simulink model "momentumBasedFlying"  (R2021b)
settings: Solver=FixedStepAuto  StartTime=0.0  StopTime=Config.simulationTime  FixedStep=Config.tStep  RelTol=1e-3
InitFcn:
  | cd(fileparts(which(bdroot)));
  | initMomentumBasedFlying;
StopFcn:
  | cd(fileparts(which(bdroot)));
  | stopMomentumBasedFlying;
undefined symbols (not defined in the file or in its folder): biasVectorConstraint_feet, Config, confVisualizer, ConstraintMatrix_feet, DiscIntNeverNeededParam, jets_config
libraries: WBToolboxLibrary x75
(part 1 of 4)
settings Model: NumberOfSteps=50  Creator=gnava  LastModifiedBy=tonhu
settings SolverCC: AlgebraicLoopSolver=LineSearch
settings DataIOCC: ReturnWorkspaceOutputs=off
settings OptimizationCC: BlockReduction=off  DefaultParameterBehavior=Inlined  BufferReuse=off
settings DebuggingCC: PregeneratedLibrarySubsystemCodeDiagnostic=none  SFMachineParentedDataDiag=warning  ArithmeticOperatorsInVariantConditions=warning
settings SFSimCC: SimUseLocalCustomCode=off  CustomCodeUndefinedFunction=UseInterfaceOnly
settings RTWCC: RTWUseLocalCustomCode=off

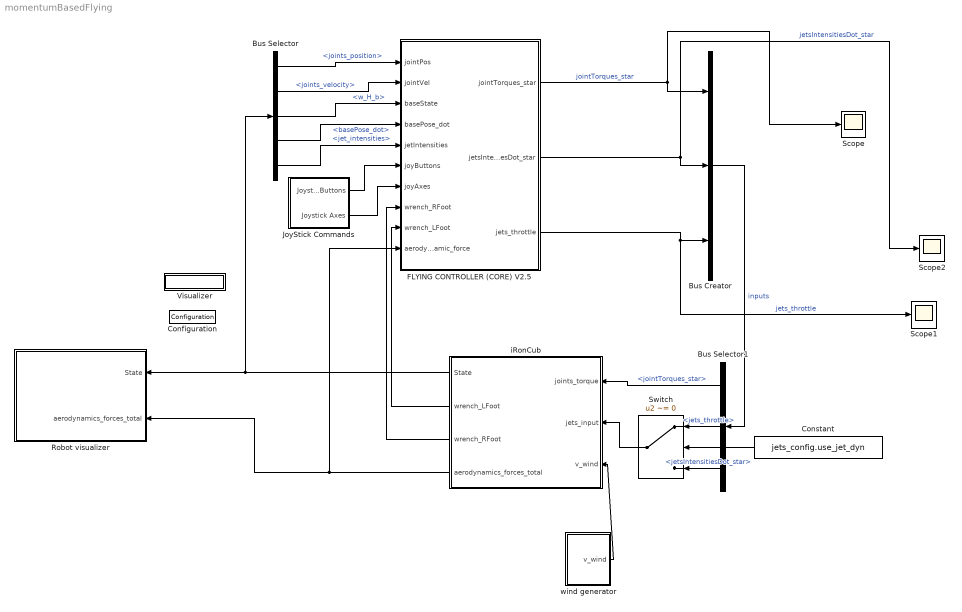
== system momentumBasedFlying ==
  Bus Creator : BusCreator  Inputs=3
  Bus Selector : BusSelector  OutputSignals=joints_position,joints_velocity,w_H_b,basePose_dot,jet_intensities
  Bus Selector1 : BusSelector  OutputSignals=jointTorques_star,jets_throttle,jetsIntensitiesDot_star
  Configuration : WBToolboxLibrary/Utilities/Configuration  ConfigSource=Workspace  ConfigObject='WBTConfigRobot'
      settings: SourceProductName=WholeBodyToolbox
  Constant : Constant  Value=jets_config.use_jet_dyn
  FLYING CONTROLLER (CORE) V2.5 : Subsystem  SystemSampleTime=0.01
  JoyStick Commands : Subsystem
  Robot visualizer : Subsystem  TreatAsAtomicUnit=on  SystemSampleTime=confVisualizer.tStep
  Scope : Scope
  Scope1 : Scope
  Scope2 : Scope
  Switch : Switch  Criteria=u2 ~= 0
  Visualizer : Subsystem
      mask Display: disp('VISUALIZER')
  iRonCub : Subsystem  SystemSampleTime=0.001
  wind generator : Subsystem
  wires:
  JoyStick Commands/1(Joystick Buttons) -> FLYING CONTROLLER (CORE) V2.5/6(joyButtons)
  JoyStick Commands/2(Joystick Axes) -> FLYING CONTROLLER (CORE) V2.5/7(joyAxes)
  iRonCub/1(State) -> Bus Selector/1, Robot visualizer/1(State)
  Bus Selector/1 -> FLYING CONTROLLER (CORE) V2.5/1(jointPos)  "<joints_position>"
  Bus Selector/2 -> FLYING CONTROLLER (CORE) V2.5/2(jointVel)  "<joints_velocity>"
  Bus Selector/3 -> FLYING CONTROLLER (CORE) V2.5/3(baseState)  "<w_H_b>"
  Bus Selector/4 -> FLYING CONTROLLER (CORE) V2.5/4("basePose_dot ")  "<basePose_dot>"
  Bus Selector/5 -> FLYING CONTROLLER (CORE) V2.5/5(jetIntensities)  "<jet_intensities>"
  Bus Creator/1 -> Bus Selector1/1  "inputs"
  FLYING CONTROLLER (CORE) V2.5/2(jetsIntensitiesDot_star) -> Scope2/1, Bus Creator/2  "jetsIntensitiesDot_star"
  FLYING CONTROLLER (CORE) V2.5/1(jointTorques_star) -> Scope/1, Bus Creator/1  "jointTorques_star"
  Bus Selector1/1 -> iRonCub/1(joints_torque)  "<jointTorques_star>"
  FLYING CONTROLLER (CORE) V2.5/3(jets_throttle) -> Scope1/1, Bus Creator/3  "jets_throttle"
  iRonCub/2(wrench_LFoot) -> FLYING CONTROLLER (CORE) V2.5/9(wrench_LFoot)
  iRonCub/3(wrench_RFoot) -> FLYING CONTROLLER (CORE) V2.5/8(wrench_RFoot)
  Switch/1 -> iRonCub/2(jets_input)
  Constant/1 -> Switch/2
  Bus Selector1/2 -> Switch/1  "<jets_throttle>"
  Bus Selector1/3 -> Switch/3  "<jetsIntensitiesDot_star>"
  iRonCub/4(aerodynamics_forces_total) -> FLYING CONTROLLER (CORE) V2.5/10(aerodynamic_force), Robot visualizer/2(aerodynamics_forces_total)
  wind generator/1(v_wind) -> iRonCub/3(v_wind)

== system momentumBasedFlying/FLYING CONTROLLER (CORE) V2.5 ==
  jointPos : Inport
  jointVel : Inport  Port=2
  baseState : Inport  Port=3
  "basePose_dot " : Inport  Port=4
  jetIntensities : Inport  Port=5
  joyButtons : Inport  Port=6
  joyAxes : Inport  Port=7
  wrench_RFoot : Inport  Port=8
  wrench_LFoot : Inport  Port=9
  aerodynamic_force : Inport  Port=10
  Dynamics and Kinematics : Subsystem
  Flight Controller RAL-HUMANOIDS V3.1- Aerodynamic Effects Compensation : Subsystem  mask{Parameter1=Config}
      mask prompts: Parameter1 "Specify the parameters struct"
      mask DialogControl DescGroupVar Prompt: Flight Controller RAL-HUMANOIDS
      mask DialogControl DescTextVar Prompt: This block implements the momentum-based flight controller decribed in RAL 2018 and HUMANOIDS 2018 papers.
      mask DialogControl Control3 Prompt: References:
      mask DialogControl Control5 Prompt: RAL 2018 paper
      mask DialogControl Control5 Callback: web https://ieeexplore.ieee.org/document/7997895
      mask DialogControl Control6 Prompt: HUMANOIDS 2018 paper
      mask DialogControl Control6 Callback: web https://ieeexplore.ieee.org/document/8624985
  Flying State Machine : Subsystem
  Get System State : Subsystem
  jointTorques_star : Outport  VectorParamsAs1DForOutWhenUnconnected=off
  jetsIntensitiesDot_star : Outport  Port=2  VectorParamsAs1DForOutWhenUnconnected=off
  jets_throttle : Outport  Port=3
  wires:
  wrench_LFoot/1 -> Get System State/6(wrench_LFoot)
  Get System State/1(systemState) -> Flight Controller RAL-HUMANOIDS V3.1- Aerodynamic Effects Compensation/3(systemState), Flying State Machine/3(systemState), Dynamics and Kinematics/1(systemState)
  joyButtons/1 -> Flying State Machine/1(joyButtons)
  jetIntensities/1 -> Get System State/7(jetIntensities)
  joyAxes/1 -> Flying State Machine/2(joyAxes)
  jointVel/1 -> Get System State/2(jointVel)
  jointPos/1 -> Get System State/1(jointPos)
  wrench_RFoot/1 -> Get System State/5(wrench_RFoot)
  baseState/1 -> Get System State/3(basePose)
  "basePose_dot "/1 -> Get System State/4("basePose_dot ")
  Flying State Machine/1(stateMachineQuantities) -> Flight Controller RAL-HUMANOIDS V3.1- Aerodynamic Effects Compensation/1(stateMachineQuantitites)
  Flying State Machine/2(gainsAndReferences) -> Flight Controller RAL-HUMANOIDS V3.1- Aerodynamic Effects Compensation/2(gainsAndReferences)
  Dynamics and Kinematics/1(kinematics) -> Flight Controller RAL-HUMANOIDS V3.1- Aerodynamic Effects Compensation/4(kinematics)
  Dynamics and Kinematics/2(dynamics) -> Flight Controller RAL-HUMANOIDS V3.1- Aerodynamic Effects Compensation/5(dynamics)
  Flight Controller RAL-HUMANOIDS V3.1- Aerodynamic Effects Compensation/1(jointTorques_star) -> jointTorques_star/1
  Flight Controller RAL-HUMANOIDS V3.1- Aerodynamic Effects Compensation/2(jetsIntensitiesDot_star) -> jetsIntensitiesDot_star/1
  Flight Controller RAL-HUMANOIDS V3.1- Aerodynamic Effects Compensation/3(jets_throttle) -> jets_throttle/1
  aerodynamic_force/1 -> Flight Controller RAL-HUMANOIDS V3.1- Aerodynamic Effects Compensation/6(aerodynamic_force)

== system momentumBasedFlying/JoyStick Commands ==
  Constant : Constant  Commented=on  Value=Config.USE_NATIVE_GUI
  Input_GUI : Constant  Value=0
  JoyStick-flightGUI Commands : Subsystem  AncestorBlock=momentum_flight_control_sublib/JoyStick-flightGUI Commands  mask{Parameter1=Config}
      mask prompts: Parameter1 "Specify the parameters struct"
      mask DialogControl DescGroupVar Prompt: Joystick/flightGUI Commands
      mask DialogControl DescTextVar Prompt: Generates commands for the flight state machine. Commands are provided by the user either using a joypad or with the native GUI.
  Joystick Axes_port : WBToolboxLibrary/Utilities/YarpRead  Commented=on  portName=Ports.JOYSTICK_AXIS  signalSize=6  timeout=0.5  blocking=off  timestamp=off  autoconnect=on  errorOnConnection=off
      settings: SourceProductName=WholeBodyToolbox
  Joystick Buttons_port : WBToolboxLibrary/Utilities/YarpRead  Commented=on  portName=Ports.JOYSTICK_BUTTONS  signalSize=24  timeout=0.5  blocking=off  timestamp=off  autoconnect=on  errorOnConnection=off
      settings: SourceProductName=WholeBodyToolbox
  Replace Joystick with Native GUI : MATLAB Function  Commented=on  TreatAsAtomicUnit=on
  Switch1 : Switch  Commented=on  Criteria=u2 > Threshold
  Switch2 : Switch  Commented=on  Criteria=u2 > Threshold
  Joystick Buttons : Outport  VectorParamsAs1DForOutWhenUnconnected=off
  Joystick Axes : Outport  Port=2  VectorParamsAs1DForOutWhenUnconnected=off
  wires:
  Input_GUI/1 -> JoyStick-flightGUI Commands/1(INPUT_GUI)
  JoyStick-flightGUI Commands/1(Button Commands) -> Joystick Buttons/1
  JoyStick-flightGUI Commands/2(Axes Commands) -> Joystick Axes/1
  Replace Joystick with Native GUI/2(joyAxes) -> Switch2/1
  Joystick Buttons_port/1 -> Switch1/3
  Joystick Axes_port/1 -> Switch2/3
  Constant/1 -> Switch2/2, Switch1/2
  Replace Joystick with Native GUI/1(joyButtons) -> Switch1/1

== system momentumBasedFlying/Robot visualizer ==
  State : Inport
  aerodynamics_forces_total : Inport  Port=2
  Bus Selector : BusSelector  OutputSignals=w_H_b,basePose_dot,joints_position,joints_velocity,jet_intensities
  Robot Visualizer : MATLABSystem  System=RobotVisualizer_iDynTree  config=confVisualizer  SimulateUsing=Interpreted execution
      mask Type: RobotVisualizer_iDynTree
      mask Display:
      | disp(['Robot' char(10) 'Visualizer']);
      | port_label('input',1,'world_H_base');
      | port_label('input',2,'base_velocity');
      | port_label('input',3,'joints_positions');
      | port_label('input',4,'joints_velocity');
      | port_label('input',5,'jetIntensities');
      | port_label('input',6,'aerodynamics_forces_total');
  wires:
  State/1 -> Bus Selector/1
  Bus Selector/1 -> Robot Visualizer/1  "<w_H_b>"
  Bus Selector/3 -> Robot Visualizer/3  "<joints_position>"
  Bus Selector/2 -> Robot Visualizer/2  "<basePose_dot>"
  Bus Selector/4 -> Robot Visualizer/4  "<joints_velocity>"
  Bus Selector/5 -> Robot Visualizer/5  "<jet_intensities>"
  aerodynamics_forces_total/1 -> Robot Visualizer/6

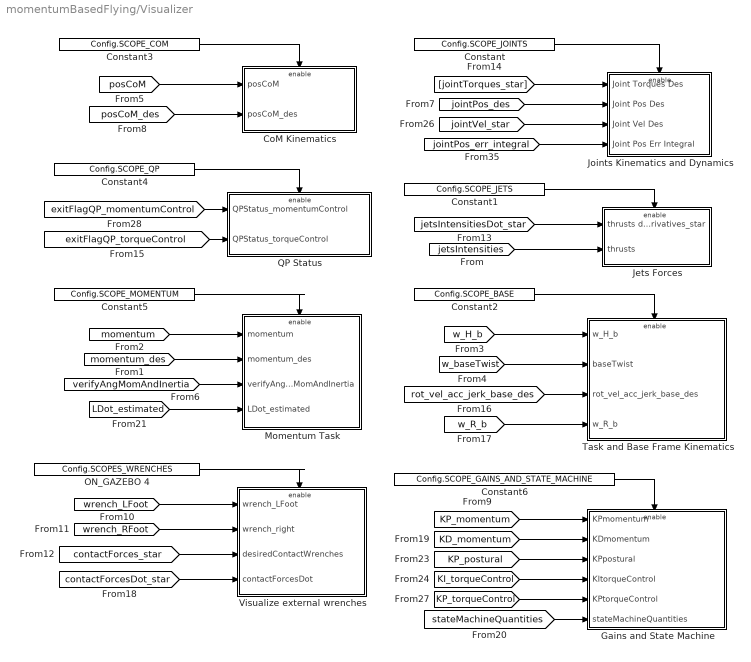
== system momentumBasedFlying/Visualizer ==
  CoM Kinematics : Subsystem
  Constant : Constant  Value=Config.SCOPE_JOINTS
  Constant1 : Constant  Value=Config.SCOPE_JETS
  Constant2 : Constant  Value=Config.SCOPE_BASE
  Constant3 : Constant  Value=Config.SCOPE_COM
  Constant4 : Constant  Value=Config.SCOPE_QP
  Constant5 : Constant  Value=Config.SCOPE_MOMENTUM
  Constant6 : Constant  Value=Config.SCOPE_GAINS_AND_STATE_MACHINE
  Gains and State Machine : Subsystem
  Jets Forces : Subsystem
  Joints Kinematics and Dynamics : Subsystem
  Momentum Task : Subsystem
  ON_GAZEBO 4 : Constant  Value=Config.SCOPES_WRENCHES
  QP Status : Subsystem
  Task and Base Frame Kinematics : Subsystem
  "Visualize external wrenches  " : Subsystem
  wires:
  [jointTorques_star] -> Joints Kinematics and Dynamics/1(Joint Torques Des)
  [jointPos_des] -> Joints Kinematics and Dynamics/2(Joint Pos Des)
  [w_H_b] -> Task and Base Frame Kinematics/1(w_H_b)
  [jointVel_star] -> Joints Kinematics and Dynamics/3(Joint Vel Des)
  Constant/1 -> Joints Kinematics and Dynamics/Enable
  [jetsIntensitiesDot_star] -> Jets Forces/1(thrusts derivatives_star)
  Constant1/1 -> Jets Forces/Enable
  [w_baseTwist] -> Task and Base Frame Kinematics/2(baseTwist)
  Constant2/1 -> Task and Base Frame Kinematics/Enable
  [momentum] -> Momentum Task/1(momentum)
  [posCoM] -> CoM Kinematics/1(posCoM)
  [posCoM_des] -> CoM Kinematics/2(posCoM_des)
  Constant3/1 -> CoM Kinematics/Enable
  [exitFlagQP_momentumControl] -> QP Status/1(QPStatus_momentumControl)
  Constant4/1 -> QP Status/Enable
  Constant5/1 -> Momentum Task/Enable
  [rot_vel_acc_jerk_base_des] -> Task and Base Frame Kinematics/3(rot_vel_acc_jerk_base_des)
  [w_R_b] -> Task and Base Frame Kinematics/4(w_R_b)
  [momentum_des] -> Momentum Task/2(momentum_des)
  [jetsIntensities] -> Jets Forces/2(thrusts)
  [verifyAngMomAndInertia] -> Momentum Task/3(verifyAngMomAndInertia)
  [wrench_LFoot] -> "Visualize external wrenches  "/1(wrench_LFoot)
  [wrench_RFoot] -> "Visualize external wrenches  "/2(wrench_right)
  ON_GAZEBO 4/1 -> "Visualize external wrenches  "/Enable
  [contactForces_star] -> "Visualize external wrenches  "/3(desiredContactWrenches)
  [exitFlagQP_torqueControl] -> QP Status/2(QPStatus_torqueControl)
  [contactForcesDot_star] -> "Visualize external wrenches  "/4(contactForcesDot)
  [LDot_estimated] -> Momentum Task/4(LDot_estimated)
  Constant6/1 -> Gains and State Machine/Enable
  [KP_momentum] -> Gains and State Machine/1(KPmomentum)
  [stateMachineQuantities] -> Gains and State Machine/6(stateMachineQuantities)
  [KD_momentum] -> Gains and State Machine/2(KDmomentum)
  [KP_postural] -> Gains and State Machine/3(KPpostural)
  [KP_torqueControl] -> Gains and State Machine/5(KPtorqueControl)
  [KI_torqueControl] -> Gains and State Machine/4(KItorqueControl)
  [jointPos_err_integral] -> Joints Kinematics and Dynamics/4(Joint Pos Err Integral)

== system momentumBasedFlying/iRonCub ==
  joints_torque : Inport
  jets_input : Inport  Port=2
  v_wind : Inport  Port=3
  Forward Dynamics : Subsystem
  State : Outport  VectorParamsAs1DForOutWhenUnconnected=off
  wrench_LFoot : Outport  Port=2
  wrench_RFoot : Outport  Port=3
  aerodynamics_forces_total : Outport  Port=4
  wires:
  jets_input/1 -> Forward Dynamics/1(jets_input)
  joints_torque/1 -> Forward Dynamics/2(joints_torque)
  Forward Dynamics/1(state) -> State/1
  Forward Dynamics/2(wrench_LFoot) -> wrench_LFoot/1
  Forward Dynamics/3(wrench_RFoot) -> wrench_RFoot/1
  Forward Dynamics/4(aerodynamics_forces_total) -> aerodynamics_forces_total/1
  v_wind/1 -> Forward Dynamics/3(v_wind)

== system momentumBasedFlying/wind generator ==
  MATLAB Function : MATLAB Function  TreatAsAtomicUnit=on
  To Workspace4 : ToWorkspace  VariableName=v_wind  SaveFormat=Timeseries  SampleTime=-1
  t : Clock
  wind : Scope
  v_wind : Outport
  wires:
  t/1 -> MATLAB Function/1(t)
  MATLAB Function/1(v_wind) -> v_wind/1, To Workspace4/1, wind/1

== system momentumBasedFlying/FLYING CONTROLLER (CORE) V2.5/Dynamics and Kinematics ==
  systemState : Inport
  Bus Creator1 : BusCreator  Inputs=5
  Bus Creator2 : BusCreator  Inputs=12
  Bus Selector : BusSelector  OutputSignals=w_H_b,jointPos,w_baseTwist,jointVel
  Dynamic Quantities : Subsystem
  Kinematic Quantities : Subsystem
  kinematics : Outport  VectorParamsAs1DForOutWhenUnconnected=off
  dynamics : Outport  Port=2  VectorParamsAs1DForOutWhenUnconnected=off
  wires:
  systemState/1 -> Bus Selector/1
  Bus Selector/1 -> Dynamic Quantities/2(w_H_b), Kinematic Quantities/1(w_H_b)  "<w_H_b>"
  Bus Selector/2 -> Dynamic Quantities/3(jointPos), Kinematic Quantities/2(jointPos)  "<jointPos>"
  Bus Selector/3 -> Dynamic Quantities/4(w_baseTwist), Kinematic Quantities/3(w_baseTwist)  "<w_baseTwist>"
  Bus Selector/4 -> Dynamic Quantities/5(jointVel), Kinematic Quantities/4(jointVel)  "<jointVel>"
  Dynamic Quantities/4(CMM) -> Bus Creator1/4  "CMM"
  Dynamic Quantities/3(L) -> Bus Creator1/3  "L"
  Dynamic Quantities/2("h ") -> Bus Creator1/2  "h"
  Dynamic Quantities/1(M) -> Bus Creator1/1  "M"
  Bus Creator1/1 -> dynamics/1
  Bus Creator2/1 -> kinematics/1
  Kinematic Quantities/1(J_jets) -> Bus Creator2/1  "J_jets"
  Kinematic Quantities/2(J_CoM) -> Bus Creator2/2  "J_CoM"
  Kinematic Quantities/3(w_R_b) -> Bus Creator2/3  "w_R_b"
  Kinematic Quantities/4(J_LFoot) -> Bus Creator2/4  "J_LFoot"
  Kinematic Quantities/5(J_RFoot) -> Bus Creator2/5  "J_RFoot"
  Kinematic Quantities/6(JDot_LFoot_nu) -> Bus Creator2/6  "JDot_LFoot_nu"
  Kinematic Quantities/7(JDot_RFoot_nu) -> Bus Creator2/7  "JDot_RFoot_nu"
  Kinematic Quantities/8(w_H_LFoot) -> Bus Creator2/8  "w_H_LFoot"
  Kinematic Quantities/9(w_H_RFoot) -> Bus Creator2/9  "w_H_RFoot"
  Kinematic Quantities/10(matrixOfJetsAxes) -> Bus Creator2/10  "matrixOfJetAxes"
  Kinematic Quantities/11(matrixOfJetsArms) -> Bus Creator2/11  "matrixOfJetsArms"
  Kinematic Quantities/12(posCoM) -> Bus Creator2/12, Dynamic Quantities/1(posCoM)  "posCoM"
  Dynamic Quantities/5(w_I_c) -> Bus Creator1/5  "w_I_c"

== system momentumBasedFlying/FLYING CONTROLLER (CORE) V2.5/Flight Controller RAL-HUMANOIDS V3.1- Aerodynamic Effects Compensation ==
  stateMachineQuantitites : Inport
  gainsAndReferences : Inport  Port=2
  systemState : Inport  Port=3
  kinematics : Inport  Port=4
  dynamics : Inport  Port=5
  aerodynamic_force : Inport  Port=6
  Joint Torque Control for Flying : Subsystem
  Momentum Control for Flying : Subsystem
  jointTorques_star : Outport  VectorParamsAs1DForOutWhenUnconnected=off
  jetsIntensitiesDot_star : Outport  Port=2  VectorParamsAs1DForOutWhenUnconnected=off
  jets_throttle : Outport  Port=3
  wires:
  Momentum Control for Flying/1(jointVel_star) -> Joint Torque Control for Flying/1(jointVel_star)
  Momentum Control for Flying/3(jetsIntensitiesDot_star) -> jetsIntensitiesDot_star/1
  Momentum Control for Flying/2(contactForces_star) -> Joint Torque Control for Flying/2(contactForces_star)
  dynamics/1 -> Momentum Control for Flying/5(dynamics), Joint Torque Control for Flying/7(dynamics)
  kinematics/1 -> Momentum Control for Flying/4(kinematics), Joint Torque Control for Flying/6(kinematics)
  systemState/1 -> Momentum Control for Flying/3(systemState), Joint Torque Control for Flying/5(systemState)
  gainsAndReferences/1 -> Momentum Control for Flying/2(gainsAndReferences), Joint Torque Control for Flying/4(gainsAndReferences)
  stateMachineQuantitites/1 -> Momentum Control for Flying/1(stateMachineQuantitites), Joint Torque Control for Flying/3(stateMachineQuantitites)
  Momentum Control for Flying/4("jets_throttle ") -> jets_throttle/1
  aerodynamic_force/1 -> Momentum Control for Flying/6(aerodynamic_force), Joint Torque Control for Flying/8(aerodynamic_force)
  Joint Torque Control for Flying/1(jointTorques_star) -> jointTorques_star/1

== system momentumBasedFlying/FLYING CONTROLLER (CORE) V2.5/Flying State Machine ==
  joyButtons : Inport
  joyAxes : Inport  Port=2
  systemState : Inport  Port=3
  Bus Selector : BusSelector  OutputSignals=jointPos
  Compute Gains And References : Subsystem
  Take Off/Landing State Detector : Subsystem
  stateMachineQuantities : Outport  VectorParamsAs1DForOutWhenUnconnected=off
  gainsAndReferences : Outport  Port=2  VectorParamsAs1DForOutWhenUnconnected=off
  wires:
  systemState/1 -> Take Off/Landing State Detector/1(systemState), Compute Gains And References/3(systemState), Bus Selector/1
  joyButtons/1 -> Take Off/Landing State Detector/2(joyButtons), Compute Gains And References/2(joyButtons)
  joyAxes/1 -> Compute Gains And References/1(joyAxes)
  Compute Gains And References/1(gainsAndReferences) -> gainsAndReferences/1
  Bus Selector/1 -> Compute Gains And References/4(jointPos)  "<jointPos>"
  Take Off/Landing State Detector/1(stateMachineQuantities) -> stateMachineQuantities/1, Compute Gains And References/5(stateMachineQuantities)

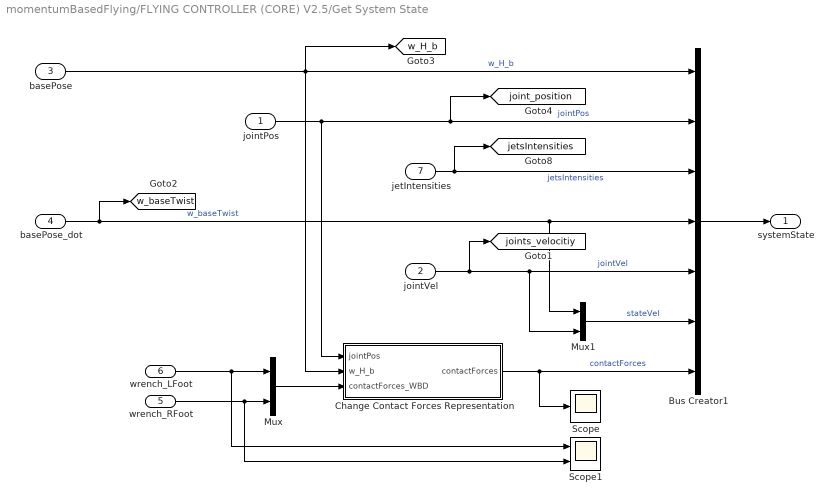
== system momentumBasedFlying/FLYING CONTROLLER (CORE) V2.5/Get System State ==
  jointPos : Inport
  jointVel : Inport  Port=2
  basePose : Inport  Port=3
  "basePose_dot " : Inport  Port=4
  wrench_RFoot : Inport  Port=5
  wrench_LFoot : Inport  Port=6
  jetIntensities : Inport  Port=7
  Bus Creator1 : BusCreator  Inputs=7
  Change Contact Forces Representation : Subsystem
  Mux : Mux  Inputs=2
  Mux1 : Mux  Inputs=2
  Scope : Scope
  Scope1 : Scope  NumInputPorts=2
  systemState : Outport  VectorParamsAs1DForOutWhenUnconnected=off
  tag scope: jetsIntensities=global, joint_position=global, joints_velocitiy=global, w_H_b=global, w_baseTwist=global
  wires:
  wrench_LFoot/1 -> Scope1/1, Mux/1
  wrench_RFoot/1 -> Scope1/2, Mux/2
  Mux/1 -> Change Contact Forces Representation/3(contactForces_WBD)
  Change Contact Forces Representation/1(contactForces) -> Scope/1, Bus Creator1/7  "contactForces"
  jointVel/1 -> [joints_velocitiy], Mux1/2, Bus Creator1/5  "jointVel"
  Bus Creator1/1 -> systemState/1
  jetIntensities/1 -> [jetsIntensities], Bus Creator1/3  "jetsIntensities"
  Mux1/1 -> Bus Creator1/6  "stateVel"
  "basePose_dot "/1 -> [w_baseTwist], Mux1/1, Bus Creator1/4  "w_baseTwist"
  basePose/1 -> Change Contact Forces Representation/2(w_H_b), [w_H_b], Bus Creator1/1  "w_H_b"
  jointPos/1 -> [joint_position], Bus Creator1/2, Change Contact Forces Representation/1(jointPos)  "jointPos"

== system momentumBasedFlying/JoyStick Commands/JoyStick-flightGUI Commands ==
  INPUT_GUI : Inport
  Replace Joystick with Native GUI : MATLAB Function  TreatAsAtomicUnit=on
  Button Commands : Outport  VectorParamsAs1DForOutWhenUnconnected=off
  Axes Commands : Outport  Port=2  VectorParamsAs1DForOutWhenUnconnected=off
  wires:
  Replace Joystick with Native GUI/2(joyAxes) -> Axes Commands/1
  Replace Joystick with Native GUI/1(joyButtons) -> Button Commands/1
  INPUT_GUI/1 -> Replace Joystick with Native GUI/1(gui_input)

== system momentumBasedFlying/Visualizer/CoM Kinematics ==
  posCoM : Inport
  posCoM_des : Inport  Port=2
  Enable : EnablePort
  CoM position : Scope  NumInputPorts=3
  CoM position desired : Scope  NumInputPorts=3
  CoM position error : Scope  NumInputPorts=3
  Demux1 : Demux  Outputs=3
  Demux2 : Demux  Outputs=3
  Demux8 : Demux  Outputs=3
  Mux : Mux  Inputs=2
  Mux1 : Mux  Inputs=2
  Mux2 : Mux  Inputs=2
  Sum : Sum  Inputs=+-|
  Task CoM combined : Scope  NumInputPorts=3
  wires:
  posCoM/1 -> Sum/1, Demux8/1
  posCoM_des/1 -> Sum/2, Demux1/1
  Sum/1 -> Demux2/1
  Demux2/3 -> CoM position error/3  "CoM_z"
  Demux2/2 -> CoM position error/2  "CoM_y"
  Demux2/1 -> CoM position error/1  "CoM_x"
  Demux8/2 -> CoM position/2, Mux1/1  "yCoM"
  Demux1/2 -> Mux1/2, CoM position desired/2  "yCoM des"
  Mux2/1 -> Task CoM combined/3
  Demux8/1 -> CoM position/1, Mux/1  "xCoM"
  Demux8/3 -> CoM position/3, Mux2/1  "zCoM"
  Mux1/1 -> Task CoM combined/2
  Demux1/1 -> CoM position desired/1, Mux/2  "xCoM des"
  Demux1/3 -> CoM position desired/3, Mux2/2  "zCoM des"
  Mux/1 -> Task CoM combined/1

== system momentumBasedFlying/Visualizer/Gains and State Machine ==
  KPmomentum : Inport
  KDmomentum : Inport  Port=2
  KPpostural : Inport  Port=3
  KItorqueControl : Inport  Port=4
  KPtorqueControl : Inport  Port=5
  stateMachineQuantities : Inport  Port=6
  Enable : EnablePort
  Bus Selector1 : BusSelector  OutputSignals=decreaseMaxFootVerticalForce,increaseMinFootVerticalForce,feetContactIsActive,robotIsLanded,oneFootIsInContact
  Feet Are in Contact : Scope
  KD_momentum : Scope
  KI_torqueControl : Scope
  KP_momentum : Scope
  KP_postural : Scope
  KP_torqueControl : Scope
  One Foot Is In Contact : Scope
  Robot Is Landed : Scope
  Start Flying Procedure : Scope
  Start Landing Procedure : Scope
  wires:
  stateMachineQuantities/1 -> Bus Selector1/1
  Bus Selector1/1 -> Start Flying Procedure/1  "<decreaseMaxFootVerticalForce>"
  Bus Selector1/2 -> Start Landing Procedure/1  "<increaseMinFootVerticalForce>"
  Bus Selector1/3 -> Feet Are in Contact/1  "<feetContactIsActive>"
  KPmomentum/1 -> KP_momentum/1
  KDmomentum/1 -> KD_momentum/1
  KPpostural/1 -> KP_postural/1
  KItorqueControl/1 -> KI_torqueControl/1
  KPtorqueControl/1 -> KP_torqueControl/1
  Bus Selector1/4 -> Robot Is Landed/1  "<robotIsLanded>"
  Bus Selector1/5 -> One Foot Is In Contact/1  "<oneFootIsInContact>"

== system momentumBasedFlying/Visualizer/Jets Forces ==
  thrusts derivatives_star : Inport
  thrusts : Inport  Port=2
  Enable : EnablePort
  thrust : Scope
  thrust derivatives_star : Scope
  wires:
  thrusts derivatives_star/1 -> thrust derivatives_star/1
  thrusts/1 -> thrust/1

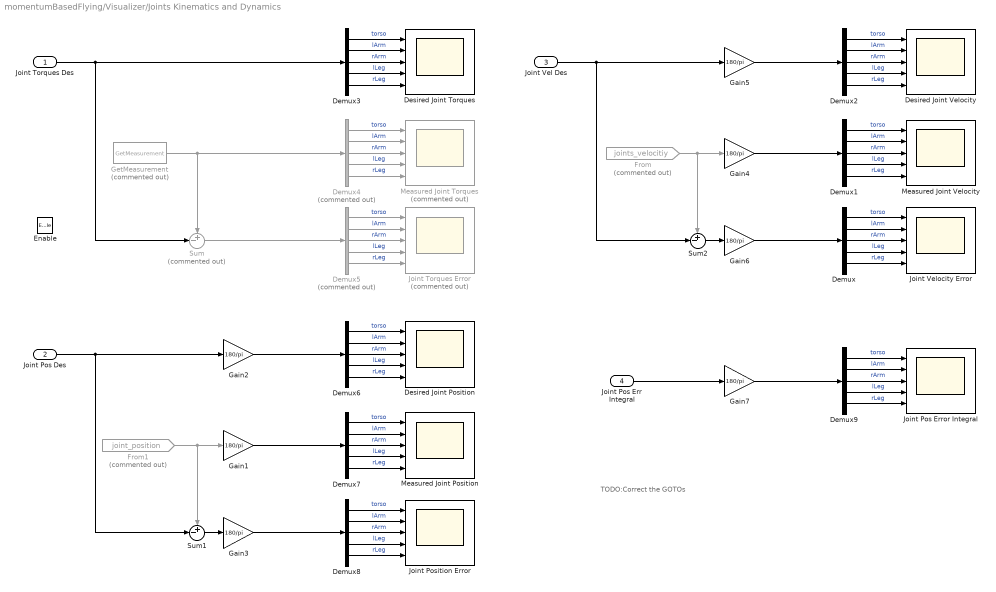
== system momentumBasedFlying/Visualizer/Joints Kinematics and Dynamics ==
  note: TODO:Correct the GOTOs
  Joint Torques Des : Inport
  Joint Pos Des : Inport  Port=2
  Joint Vel Des : Inport  Port=3
  Joint Pos Err Integral : Inport  Port=4
  Enable : EnablePort
  Demux{,1..3,6..9} (8 alike) : Demux  Outputs=Config.numOfJointsForEachControlboard
  Demux4 : Demux  Commented=on  Outputs=Config.numOfJointsForEachControlboard
  Demux5 : Demux  Commented=on  Outputs=Config.numOfJointsForEachControlboard
  Desired Joint Position : Scope  NumInputPorts=5
  Desired Joint Torques : Scope  NumInputPorts=5
  Desired Joint Velocity : Scope  NumInputPorts=5
  From : From  Commented=on  GotoTag=joints_velocitiy  TagVisibility=global
  From1 : From  Commented=on  GotoTag=joint_position  TagVisibility=global
  Gain{1..7} (7 alike) : Gain  Gain=180/pi
  GetMeasurement : WBToolboxLibrary/States/GetMeasurement  Commented=on  measuredType=Joints Torque
      settings: SourceProductName=WholeBodyToolbox
  Joint Pos Error Integral : Scope  NumInputPorts=5
  Joint Position Error : Scope  NumInputPorts=5
  Joint Torques Error : Scope  Commented=on  NumInputPorts=5
  Joint Velocity Error : Scope  NumInputPorts=5
  Measured Joint Position : Scope  NumInputPorts=5
  Measured Joint Torques : Scope  Commented=on  NumInputPorts=5
  Measured Joint Velocity : Scope  NumInputPorts=5
  Sum : Sum  Commented=on  Inputs=+-|
  Sum1 : Sum  Inputs=+-|
  Sum2 : Sum  Inputs=+-|
  wires:
  Demux5/3 -> Joint Torques Error/3  "rArm"
  Demux5/4 -> Joint Torques Error/4  "lLeg"
  Demux5/5 -> Joint Torques Error/5  "rLeg"
  Sum/1 -> Demux5/1
  Demux5/1 -> Joint Torques Error/1  "torso"
  Demux5/2 -> Joint Torques Error/2  "lArm"
  GetMeasurement/1 -> Demux4/1, Sum/1
  Demux4/3 -> Measured Joint Torques/3  "rArm"
  Demux4/2 -> Measured Joint Torques/2  "lArm"
  Demux4/5 -> Measured Joint Torques/5  "rLeg"
  Demux4/4 -> Measured Joint Torques/4  "lLeg"
  Demux4/1 -> Measured Joint Torques/1  "torso"
  Demux3/1 -> Desired Joint Torques/1  "torso"
  Demux3/5 -> Desired Joint Torques/5  "rLeg"
  Joint Torques Des/1 -> Demux3/1, Sum/2
  Demux3/3 -> Desired Joint Torques/3  "rArm"
  Demux3/2 -> Desired Joint Torques/2  "lArm"
  Demux3/4 -> Desired Joint Torques/4  "lLeg"
  Demux7/4 -> Measured Joint Position/4  "lLeg"
  Demux7/2 -> Measured Joint Position/2  "lArm"
  Joint Pos Des/1 -> Sum1/2, Gain2/1
  Demux8/2 -> Joint Position Error/2  "lArm"
  Sum1/1 -> Gain3/1
  Demux7/1 -> Measured Joint Position/1  "torso"
  Demux8/5 -> Joint Position Error/5  "rLeg"
  From1/1 -> Sum1/1, Gain1/1
  Demux8/4 -> Joint Position Error/4  "lLeg"
  Demux6/1 -> Desired Joint Position/1  "torso"
  Demux8/3 -> Joint Position Error/3  "rArm"
  Demux6/2 -> Desired Joint Position/2  "lArm"
  Demux6/4 -> Desired Joint Position/4  "lLeg"
  Demux7/5 -> Measured Joint Position/5  "rLeg"
  Demux6/5 -> Desired Joint Position/5  "rLeg"
  Demux8/1 -> Joint Position Error/1  "torso"
  Demux7/3 -> Measured Joint Position/3  "rArm"
  Demux6/3 -> Desired Joint Position/3  "rArm"
  Gain1/1 -> Demux7/1
  Gain2/1 -> Demux6/1
  Gain3/1 -> Demux8/1
  Joint Vel Des/1 -> Sum2/2, Gain5/1
  Demux2/3 -> Desired Joint Velocity/3  "rArm"
  Demux/3 -> Joint Velocity Error/3  "rArm"
  Demux2/1 -> Desired Joint Velocity/1  "torso"
  Demux2/5 -> Desired Joint Velocity/5  "rLeg"
  Demux2/4 -> Desired Joint Velocity/4  "lLeg"
  Demux1/5 -> Measured Joint Velocity/5  "rLeg"
  Demux1/1 -> Measured Joint Velocity/1  "torso"
  Demux/5 -> Joint Velocity Error/5  "rLeg"
  Gain4/1 -> Demux1/1
  Demux/2 -> Joint Velocity Error/2  "lArm"
  Demux/1 -> Joint Velocity Error/1  "torso"
  Demux/4 -> Joint Velocity Error/4  "lLeg"
  Sum2/1 -> Gain6/1
  Demux1/2 -> Measured Joint Velocity/2  "lArm"
  Demux1/4 -> Measured Joint Velocity/4  "lLeg"
  Demux2/2 -> Desired Joint Velocity/2  "lArm"
  Demux1/3 -> Measured Joint Velocity/3  "rArm"
  Gain6/1 -> Demux/1
  Gain5/1 -> Demux2/1
  From/1 -> Sum2/1, Gain4/1
  Demux9/1 -> Joint Pos Error Integral/1  "torso"
  Demux9/5 -> Joint Pos Error Integral/5  "rLeg"
  Joint Pos Err Integral/1 -> Gain7/1
  Gain7/1 -> Demux9/1
  Demux9/3 -> Joint Pos Error Integral/3  "rArm"
  Demux9/2 -> Joint Pos Error Integral/2  "lArm"
  Demux9/4 -> Joint Pos Error Integral/4  "lLeg"

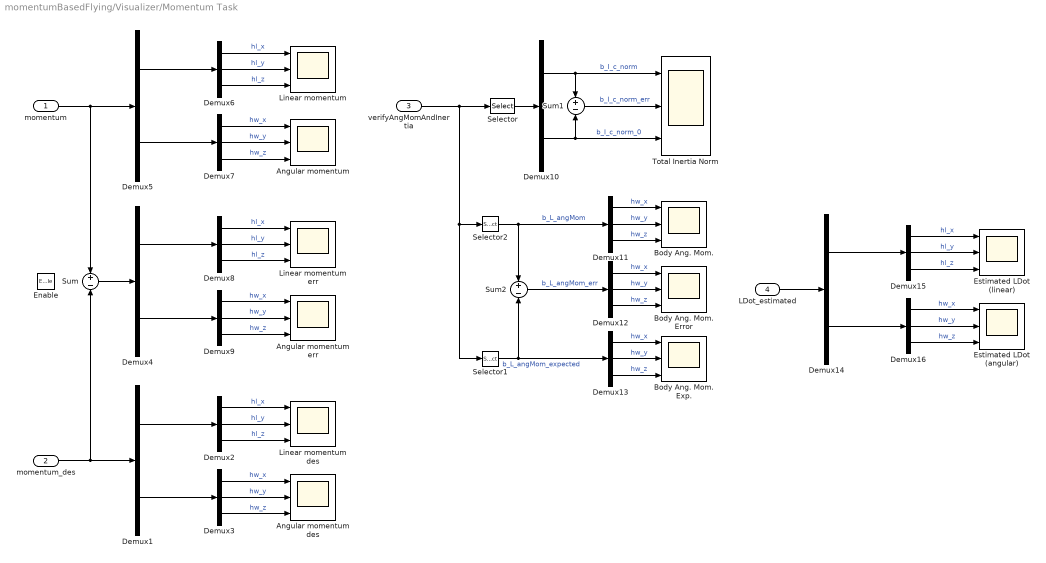
== system momentumBasedFlying/Visualizer/Momentum Task ==
  momentum : Inport
  momentum_des : Inport  Port=2
  verifyAngMomAndInertia : Inport  Port=3
  LDot_estimated : Inport  Port=4
  Enable : EnablePort
  Angular momentum : Scope  NumInputPorts=3
  Angular momentum des : Scope  NumInputPorts=3
  Angular momentum err : Scope  NumInputPorts=3
  Body Ang. Mom. : Scope  NumInputPorts=3
  Body Ang. Mom. Error : Scope  NumInputPorts=3
  Body Ang. Mom. Exp. : Scope  NumInputPorts=3
  Demux{1,4..5,10,14} (5 alike) : Demux  Outputs=2
  Demux{2..3,6..9,11..13,15..16} (11 alike) : Demux  Outputs=3
  Estimated LDot (angular) : Scope  NumInputPorts=3
  Estimated LDot (linear) : Scope  NumInputPorts=3
  Linear momentum : Scope  NumInputPorts=3
  Linear momentum des : Scope  NumInputPorts=3
  Linear momentum err : Scope  NumInputPorts=3
  Selector : Selector  NumberOfDimensions=2  InputPortWidth=3  IndexOptions=Index vector (dialog),Index vector (dialog)  Indices=[1],[1 2]  OutputSizes=1,1
  Selector1 : Selector  NumberOfDimensions=2  InputPortWidth=3  IndexOptions=Index vector (dialog),Index vector (dialog)  Indices=[2 3 4],[2]  OutputSizes=1,1
  Selector2 : Selector  NumberOfDimensions=2  InputPortWidth=3  IndexOptions=Index vector (dialog),Index vector (dialog)  Indices=[2 3 4],[1]  OutputSizes=1,1
  Sum : Sum  Inputs=+|-
  Sum1 : Sum  Inputs=+|-
  Sum2 : Sum  Inputs=+|-
  Total Inertia Norm : Scope  NumInputPorts=3
  wires:
  Demux6/1 -> Linear momentum/1  "hl_x"
  Demux6/3 -> Linear momentum/3  "hl_z"
  Demux5/2 -> Demux7/1
  Demux6/2 -> Linear momentum/2  "hl_y"
  Demux5/1 -> Demux6/1
  Demux7/1 -> Angular momentum/1  "hw_x"
  Demux7/3 -> Angular momentum/3  "hw_z"
  Demux7/2 -> Angular momentum/2  "hw_y"
  momentum/1 -> Sum/1, Demux5/1
  Demux3/2 -> Angular momentum des/2  "hw_y"
  Demux3/1 -> Angular momentum des/1  "hw_x"
  Demux2/3 -> Linear momentum des/3  "hl_z"
  Demux2/1 -> Linear momentum des/1  "hl_x"
  Demux1/2 -> Demux3/1
  Demux1/1 -> Demux2/1
  Demux3/3 -> Angular momentum des/3  "hw_z"
  Demux2/2 -> Linear momentum des/2  "hl_y"
  momentum_des/1 -> Sum/2, Demux1/1
  Demux9/2 -> Angular momentum err/2  "hw_y"
  Demux9/1 -> Angular momentum err/1  "hw_x"
  Demux8/3 -> Linear momentum err/3  "hl_z"
  Demux8/1 -> Linear momentum err/1  "hl_x"
  Demux4/2 -> Demux9/1
  Demux4/1 -> Demux8/1
  Demux9/3 -> Angular momentum err/3  "hw_z"
  Demux8/2 -> Linear momentum err/2  "hl_y"
  Sum/1 -> Demux4/1
  verifyAngMomAndInertia/1 -> Selector/1, Selector1/1, Selector2/1
  Selector/1 -> Demux10/1
  Demux10/1 -> Total Inertia Norm/1, Sum1/1  "b_I_c_norm"
  Demux10/2 -> Total Inertia Norm/3, Sum1/2  "b_I_c_norm_0"
  Sum1/1 -> Total Inertia Norm/2  "b_I_c_norm_err"
  Selector2/1 -> Demux11/1, Sum2/1  "b_L_angMom"
  Demux11/2 -> Body Ang. Mom./2  "hw_y"
  Demux11/3 -> Body Ang. Mom./3  "hw_z"
  Demux11/1 -> Body Ang. Mom./1  "hw_x"
  Demux12/2 -> Body Ang. Mom. Error/2  "hw_y"
  Sum2/1 -> Demux12/1  "b_L_angMom_err"
  Demux12/3 -> Body Ang. Mom. Error/3  "hw_z"
  Demux12/1 -> Body Ang. Mom. Error/1  "hw_x"
  Demux13/2 -> Body Ang. Mom. Exp./2  "hw_y"
  Selector1/1 -> Sum2/2, Demux13/1  "b_L_angMom_expected"
  Demux13/3 -> Body Ang. Mom. Exp./3  "hw_z"
  Demux13/1 -> Body Ang. Mom. Exp./1  "hw_x"
  LDot_estimated/1 -> Demux14/1
  Demux15/3 -> Estimated LDot (linear)/3  "hl_z"
  Demux16/2 -> Estimated LDot (angular)/2  "hw_y"
  Demux14/1 -> Demux15/1
  Demux14/2 -> Demux16/1
  Demux15/2 -> Estimated LDot (linear)/2  "hl_y"
  Demux15/1 -> Estimated LDot (linear)/1  "hl_x"
  Demux16/1 -> Estimated LDot (angular)/1  "hw_x"
  Demux16/3 -> Estimated LDot (angular)/3  "hw_z"

== system momentumBasedFlying/Visualizer/QP Status ==
  QPStatus_momentumControl : Inport
  QPStatus_torqueControl : Inport  Port=2
  Enable : EnablePort
  QP momentum : Scope
  QP torques : Scope
  wires:
  QPStatus_momentumControl/1 -> QP momentum/1
  QPStatus_torqueControl/1 -> QP torques/1

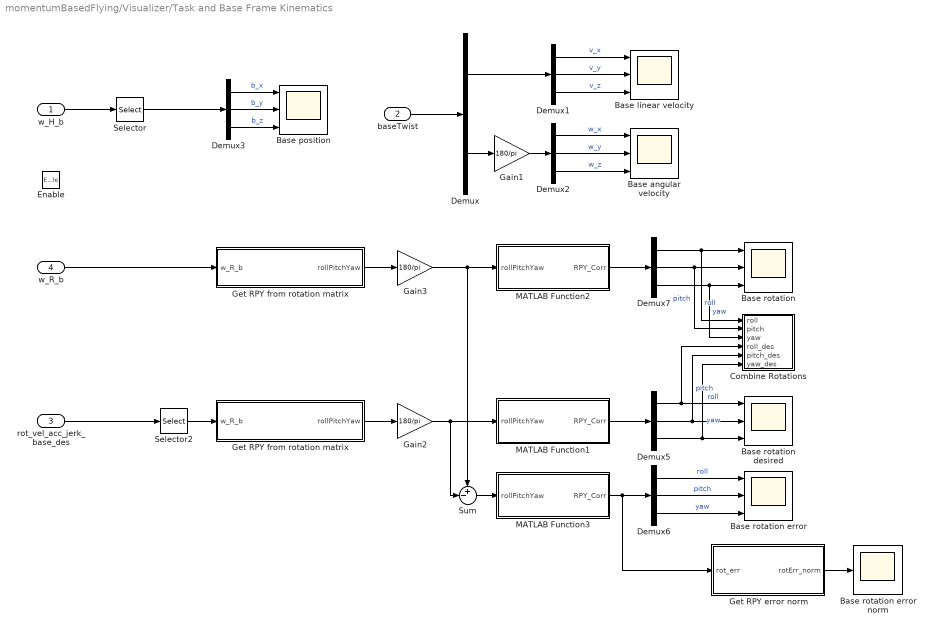
== system momentumBasedFlying/Visualizer/Task and Base Frame Kinematics ==
  w_H_b : Inport
  baseTwist : Inport  Port=2
  rot_vel_acc_jerk_base_des : Inport  Port=3
  w_R_b : Inport  Port=4
  Enable : EnablePort
  Base angular velocity : Scope  NumInputPorts=3
  Base linear velocity : Scope  NumInputPorts=3
  Base position : Scope  NumInputPorts=3
  Base rotation : Scope  NumInputPorts=3
  Base rotation desired : Scope  NumInputPorts=3
  Base rotation error : Scope  NumInputPorts=3
  Base rotation error norm : Scope
  Combine Rotations : Subsystem
  Demux : Demux  Outputs=2
  Demux{1..3,5..7} (6 alike) : Demux  Outputs=3
  Gain1 : Gain  Gain=180/pi
  Gain2 : Gain  Gain=180/pi
  Gain3 : Gain  Gain=180/pi
  Get RPY error norm : MATLAB Function  TreatAsAtomicUnit=on
  Get RPY from rotation matrix : MATLAB Function  TreatAsAtomicUnit=on
  "Get RPY from rotation matrix " : MATLAB Function  TreatAsAtomicUnit=on
  MATLAB Function1 : MATLAB Function  TreatAsAtomicUnit=on
  MATLAB Function2 : MATLAB Function  TreatAsAtomicUnit=on
  MATLAB Function3 : MATLAB Function  TreatAsAtomicUnit=on
  Selector : Selector  NumberOfDimensions=2  InputPortWidth=3  IndexOptions=Index vector (dialog),Index vector (dialog)  Indices=[1:3],4  OutputSizes=1,1
  Selector2 : Selector  NumberOfDimensions=2  InputPortWidth=3  IndexOptions=Index vector (dialog),Index vector (dialog)  Indices=[1:3],[1:3]  OutputSizes=1,1
  Sum : Sum  Inputs=+-|
  wires:
  Demux3/1 -> Base position/1  "b_x"
  Demux3/3 -> Base position/3  "b_z"
  Demux3/2 -> Base position/2  "b_y"
  Selector/1 -> Demux3/1
  w_H_b/1 -> Selector/1
  Demux1/1 -> Base linear velocity/1  "v_x"
  Demux1/3 -> Base linear velocity/3  "v_z"
  Demux2/3 -> Base angular velocity/3  "w_z"
  Demux/2 -> Gain1/1
  Demux2/1 -> Base angular velocity/1  "w_x"
  Demux/1 -> Demux1/1
  Demux2/2 -> Base angular velocity/2  "w_y"
  Gain1/1 -> Demux2/1
  Demux1/2 -> Base linear velocity/2  "v_y"
  "Get RPY from rotation matrix "/1(rollPitchYaw) -> Gain2/1
  Demux5/1 -> Combine Rotations/4(roll_des), Base rotation desired/1  "roll"
  Gain2/1 -> MATLAB Function1/1(rollPitchYaw), Sum/2
  Demux5/2 -> Combine Rotations/5(pitch_des), Base rotation desired/2  "pitch"
  Selector2/1 -> "Get RPY from rotation matrix "/1(w_R_b)
  Demux5/3 -> Combine Rotations/6(yaw_des), Base rotation desired/3  "yaw"
  Demux6/2 -> Base rotation error/2  "pitch"
  Demux6/1 -> Base rotation error/1  "roll"
  Demux6/3 -> Base rotation error/3  "yaw"
  Sum/1 -> MATLAB Function3/1(rollPitchYaw)
  baseTwist/1 -> Demux/1
  rot_vel_acc_jerk_base_des/1 -> Selector2/1
  Gain3/1 -> MATLAB Function2/1(rollPitchYaw), Sum/1
  Demux7/2 -> Combine Rotations/2(pitch), Base rotation/2  "pitch"
  Get RPY from rotation matrix/1(rollPitchYaw) -> Gain3/1
  Demux7/1 -> Combine Rotations/1(roll), Base rotation/1  "roll"
  Demux7/3 -> Combine Rotations/3(yaw), Base rotation/3  "yaw"
  w_R_b/1 -> Get RPY from rotation matrix/1(w_R_b)
  Get RPY error norm/1(rotErr_norm) -> Base rotation error norm/1
  MATLAB Function3/1(RPY_Corr) -> Demux6/1, Get RPY error norm/1(rot_err)
  MATLAB Function1/1(RPY_Corr) -> Demux5/1
  MATLAB Function2/1(RPY_Corr) -> Demux7/1

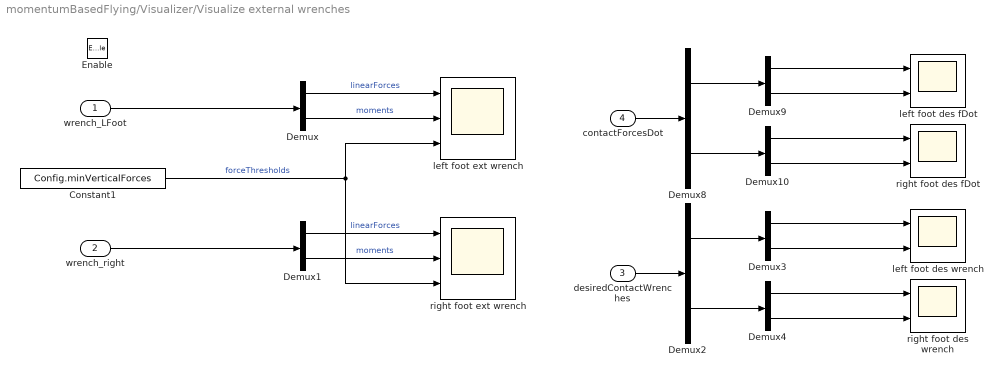
== system momentumBasedFlying/Visualizer/Visualize external wrenches   ==
  wrench_LFoot : Inport
  wrench_right : Inport  Port=2
  desiredContactWrenches : Inport  Port=3
  contactForcesDot : Inport  Port=4
  Enable : EnablePort
  Constant1 : Constant  Value=Config.minVerticalForces
  Demux{,1,3..4,9..10} (6 alike) : Demux  Outputs=[3;3]
  Demux2 : Demux  Outputs=[6;6]
  Demux8 : Demux  Outputs=[6;6]
  left foot des fDot : Scope  NumInputPorts=2
  left foot des wrench : Scope  NumInputPorts=2
  left foot ext wrench : Scope  NumInputPorts=3
  right foot des fDot : Scope  NumInputPorts=2
  right foot des wrench : Scope  NumInputPorts=2
  right foot ext wrench : Scope  NumInputPorts=3
  wires:
  Demux/1 -> left foot ext wrench/1  "linearForces"
  Demux/2 -> left foot ext wrench/2  "moments"
  Demux1/1 -> right foot ext wrench/1  "linearForces"
  Demux1/2 -> right foot ext wrench/2  "moments"
  wrench_LFoot/1 -> Demux/1
  wrench_right/1 -> Demux1/1
  desiredContactWrenches/1 -> Demux2/1
  Demux2/1 -> Demux3/1
  Demux2/2 -> Demux4/1
  Demux4/1 -> right foot des wrench/1
  Demux4/2 -> right foot des wrench/2
  Demux3/1 -> left foot des wrench/1
  Demux3/2 -> left foot des wrench/2
  Demux8/2 -> Demux10/1
  contactForcesDot/1 -> Demux8/1
  Demux10/2 -> right foot des fDot/2
  Demux8/1 -> Demux9/1
  Demux10/1 -> right foot des fDot/1
  Demux9/2 -> left foot des fDot/2
  Demux9/1 -> left foot des fDot/1
  Constant1/1 -> right foot ext wrench/3, left foot ext wrench/3  "forceThresholds"

== system momentumBasedFlying/iRonCub/Forward Dynamics ==
  jets_input : Inport
  joints_torque : Inport  Port=2
  v_wind : Inport  Port=3
  Bus Creator1 : BusCreator  Inputs=5
  Delay : Delay  DelayLength=1
  Delay1 : Delay  DelayLength=1
  MATLAB System1 : MATLABSystem  System=step_block  robot_config=robot_config  contact_config=contact_config  jets_config=jets_config  tStep=Config.tStep  aerodynamics_config=aerodynamics_config  SimulateUsing=Interpreted execution
      mask Type: step_block
      mask Display:
      | disp('step_block');
      | port_label('input',1,'jets_input');
      | port_label('input',2,'torque');
      | port_label('input',3,'v_wind');
      | port_label('output',1,'w_H_b');
      | port_label('output',2,'s');
      | port_label('output',3,'base_pose_dot');
      | port_label('output',4,'s_dot');
      | port_label('output',5,'jet_intensities');
      | port_label('output',6,'wrench_left_foot');
      | port_label('output',7,'wrench_right_foot');
      | port_label('output',8,'aerodynamic_forces_total');
      | port_label('output',9,'relative_velocity');
      | port_label('output',10,'alpha');
      | port_label('output',11,'beta');
      | port_label('output',12,'drag_force');
      | port_label('output',13,'normal_force');
  aerodynamic visualizer : Subsystem
  state : Outport
  wrench_LFoot : Outport  Port=2
  wrench_RFoot : Outport  Port=3
  aerodynamics_forces_total : Outport  Port=4
  wires:
  jets_input/1 -> Delay1/1
  joints_torque/1 -> Delay/1
  MATLAB System1/1 -> Bus Creator1/1  "w_H_b"
  MATLAB System1/2 -> Bus Creator1/2  "joints_position"
  Bus Creator1/1 -> state/1  "state"
  MATLAB System1/4 -> Bus Creator1/4  "joints_velocity"
  MATLAB System1/3 -> Bus Creator1/3  "basePose_dot"
  Delay/1 -> MATLAB System1/2
  MATLAB System1/5 -> Bus Creator1/5  "jet_intensities"
  Delay1/1 -> MATLAB System1/1
  MATLAB System1/6 -> wrench_LFoot/1  "wrench_LFoot"
  MATLAB System1/7 -> wrench_RFoot/1  "wrench_RFoot"
  MATLAB System1/10 -> aerodynamic visualizer/3(alpha)
  MATLAB System1/11 -> aerodynamic visualizer/4(beta)
  v_wind/1 -> MATLAB System1/3
  MATLAB System1/8 -> aerodynamics_forces_total/1, aerodynamic visualizer/1(aerodynamic_forces_total)
  MATLAB System1/9 -> aerodynamic visualizer/2(relative_velocity)
  MATLAB System1/12 -> aerodynamic visualizer/5(drag_force)
  MATLAB System1/13 -> aerodynamic visualizer/6(normal_force)

== system momentumBasedFlying/FLYING CONTROLLER (CORE) V2.5/Dynamics and Kinematics/Dynamic Quantities ==
  posCoM : Inport
  w_H_b : Inport  Port=2
  jointPos : Inport  Port=3
  w_baseTwist : Inport  Port=4
  jointVel : Inport  Port=5
  Compute Centroidal Inertia : Subsystem
  GetBiasForces : WBToolboxLibrary/Model/Dynamics/GetBiasForces
      settings: SourceProductName=WholeBodyToolbox
  MassMatrix : WBToolboxLibrary/Model/Dynamics/MassMatrix
      settings: SourceProductName=WholeBodyToolbox
  Momentum and CentroidalMomentum Matrix : Subsystem
  M : Outport  VectorParamsAs1DForOutWhenUnconnected=off
  "h " : Outport  Port=2  VectorParamsAs1DForOutWhenUnconnected=off
  L : Outport  Port=3  VectorParamsAs1DForOutWhenUnconnected=off
  CMM : Outport  Port=4  VectorParamsAs1DForOutWhenUnconnected=off
  w_I_c : Outport  Port=5  VectorParamsAs1DForOutWhenUnconnected=off
  tag scope: momentum=global
  wires:
  w_H_b/1 -> Momentum and CentroidalMomentum Matrix/1(w_H_b), GetBiasForces/1, Compute Centroidal Inertia/2(w_H_b), MassMatrix/1  "w_H_b"
  w_baseTwist/1 -> Momentum and CentroidalMomentum Matrix/3(w_baseTwist), GetBiasForces/3
  jointVel/1 -> Momentum and CentroidalMomentum Matrix/4(jointVel), GetBiasForces/4
  MassMatrix/1 -> Compute Centroidal Inertia/1(M), M/1
  GetBiasForces/1 -> "h "/1
  Momentum and CentroidalMomentum Matrix/2(CMM) -> CMM/1
  Momentum and CentroidalMomentum Matrix/1(L) -> L/1, [momentum]
  jointPos/1 -> GetBiasForces/2, MassMatrix/2, Momentum and CentroidalMomentum Matrix/2(jointPos)
  Compute Centroidal Inertia/1(w_I_c) -> w_I_c/1
  posCoM/1 -> Compute Centroidal Inertia/3(posCoM)  "com_pos"

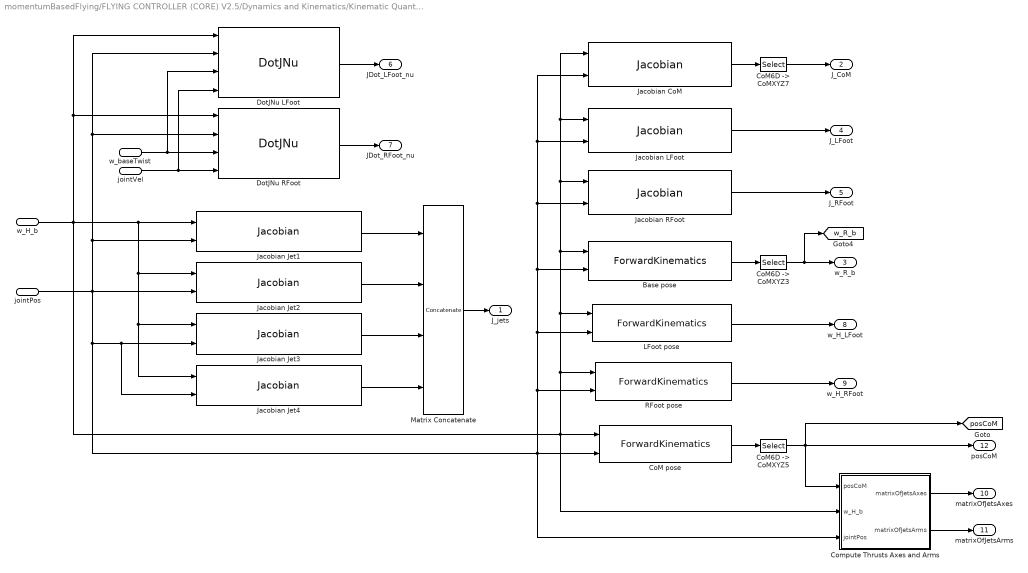
== system momentumBasedFlying/FLYING CONTROLLER (CORE) V2.5/Dynamics and Kinematics/Kinematic Quantities ==
  w_H_b : Inport
  jointPos : Inport  Port=2
  w_baseTwist : Inport  Port=3
  jointVel : Inport  Port=4
  Base pose : WBToolboxLibrary/Model/Kinematics/ForwardKinematics  frameName=Frames.BASE_LINK
      settings: SourceProductName=WholeBodyToolbox
  CoM pose : WBToolboxLibrary/Model/Kinematics/ForwardKinematics  frameName=Frames.COM_FRAME
      settings: SourceProductName=WholeBodyToolbox
  "CoM6D -> CoMXYZ3" : Selector  NumberOfDimensions=2  InputPortWidth=7  IndexOptions=Index vector (dialog),Index vector (dialog)  Indices=[1 2 3],[1 2 3]  OutputSizes=1,1
  "CoM6D -> CoMXYZ5" : Selector  NumberOfDimensions=2  InputPortWidth=7  IndexOptions=Index vector (dialog),Index vector (dialog)  Indices=[1 2 3],[4]  OutputSizes=1,1
  "CoM6D -> CoMXYZ7" : Selector  NumberOfDimensions=2  InputPortWidth=7  IndexOptions=Index vector (dialog),Index vector (dialog)  Indices=[1 2 3],[1:6+Config.N_DOF]  OutputSizes=1,1
  Compute Thrusts Axes and Arms : Subsystem
  DotJNu LFoot : WBToolboxLibrary/Model/Jacobians/DotJNu  frameName=Frames.LFOOT_FRAME
      settings: SourceProductName=WholeBodyToolbox
  DotJNu RFoot : WBToolboxLibrary/Model/Jacobians/DotJNu  frameName=Frames.RFOOT_FRAME
      settings: SourceProductName=WholeBodyToolbox
  Jacobian CoM : WBToolboxLibrary/Model/Jacobians/Jacobian  frameName=Frames.COM_FRAME
      settings: SourceProductName=WholeBodyToolbox
  Jacobian Jet1 : WBToolboxLibrary/Model/Jacobians/Jacobian  frameName=Frames.JET1_FRAME
      settings: SourceProductName=WholeBodyToolbox
  Jacobian Jet2 : WBToolboxLibrary/Model/Jacobians/Jacobian  frameName=Frames.JET2_FRAME
      settings: SourceProductName=WholeBodyToolbox
  Jacobian Jet3 : WBToolboxLibrary/Model/Jacobians/Jacobian  frameName=Frames.JET3_FRAME
      settings: SourceProductName=WholeBodyToolbox
  Jacobian Jet4 : WBToolboxLibrary/Model/Jacobians/Jacobian  frameName=Frames.JET4_FRAME
      settings: SourceProductName=WholeBodyToolbox
  Jacobian LFoot : WBToolboxLibrary/Model/Jacobians/Jacobian  frameName=Frames.LFOOT_FRAME
      settings: SourceProductName=WholeBodyToolbox
  Jacobian RFoot : WBToolboxLibrary/Model/Jacobians/Jacobian  frameName=Frames.RFOOT_FRAME
      settings: SourceProductName=WholeBodyToolbox
  LFoot pose : WBToolboxLibrary/Model/Kinematics/ForwardKinematics  frameName=Frames.LFOOT_FRAME
      settings: SourceProductName=WholeBodyToolbox
  Matrix Concatenate : Concatenate  NumInputs=4  Mode=Multidimensional array
  RFoot pose : WBToolboxLibrary/Model/Kinematics/ForwardKinematics  frameName=Frames.RFOOT_FRAME
      settings: SourceProductName=WholeBodyToolbox
  J_jets : Outport  VectorParamsAs1DForOutWhenUnconnected=off
  J_CoM : Outport  Port=2  VectorParamsAs1DForOutWhenUnconnected=off
  w_R_b : Outport  Port=3  VectorParamsAs1DForOutWhenUnconnected=off
  J_LFoot : Outport  Port=4  VectorParamsAs1DForOutWhenUnconnected=off
  J_RFoot : Outport  Port=5  VectorParamsAs1DForOutWhenUnconnected=off
  JDot_LFoot_nu : Outport  Port=6  VectorParamsAs1DForOutWhenUnconnected=off
  JDot_RFoot_nu : Outport  Port=7  VectorParamsAs1DForOutWhenUnconnected=off
  w_H_LFoot : Outport  Port=8  VectorParamsAs1DForOutWhenUnconnected=off
  w_H_RFoot : Outport  Port=9  VectorParamsAs1DForOutWhenUnconnected=off
  matrixOfJetsAxes : Outport  Port=10  VectorParamsAs1DForOutWhenUnconnected=off
  matrixOfJetsArms : Outport  Port=11  VectorParamsAs1DForOutWhenUnconnected=off
  posCoM : Outport  Port=12  VectorParamsAs1DForOutWhenUnconnected=off
  tag scope: posCoM=global, w_R_b=global
  wires:
  Matrix Concatenate/1 -> J_jets/1
  CoM pose/1 -> "CoM6D -> CoMXYZ5"/1
  "CoM6D -> CoMXYZ5"/1 -> posCoM/1, [posCoM], Compute Thrusts Axes and Arms/1(posCoM)
  w_H_b/1 -> LFoot pose/1, Base pose/1, Jacobian LFoot/1, Jacobian CoM/1, Jacobian RFoot/1, RFoot pose/1, CoM pose/1, Compute Thrusts Axes and Arms/2(w_H_b), DotJNu LFoot/1, DotJNu RFoot/1, Jacobian Jet4/1, Jacobian Jet3/1, Jacobian Jet2/1, Jacobian Jet1/1
  "CoM6D -> CoMXYZ3"/1 -> w_R_b/1, [w_R_b]
  jointPos/1 -> Jacobian Jet4/2, Jacobian Jet3/2, Compute Thrusts Axes and Arms/3(jointPos), LFoot pose/2, Jacobian RFoot/2, Jacobian LFoot/2, Jacobian CoM/2, Base pose/2, RFoot pose/2, CoM pose/2, Jacobian Jet2/2, DotJNu LFoot/2, DotJNu RFoot/2, Jacobian Jet1/2
  Jacobian CoM/1 -> "CoM6D -> CoMXYZ7"/1
  Jacobian RFoot/1 -> J_RFoot/1
  Jacobian LFoot/1 -> J_LFoot/1
  DotJNu RFoot/1 -> JDot_RFoot_nu/1
  DotJNu LFoot/1 -> JDot_LFoot_nu/1
  jointVel/1 -> DotJNu RFoot/4, DotJNu LFoot/4
  w_baseTwist/1 -> DotJNu LFoot/3, DotJNu RFoot/3
  RFoot pose/1 -> w_H_RFoot/1
  LFoot pose/1 -> w_H_LFoot/1
  Base pose/1 -> "CoM6D -> CoMXYZ3"/1
  Compute Thrusts Axes and Arms/2(matrixOfJetsArms) -> matrixOfJetsArms/1
  Compute Thrusts Axes and Arms/1(matrixOfJetsAxes) -> matrixOfJetsAxes/1
  Jacobian Jet1/1 -> Matrix Concatenate/1
  Jacobian Jet2/1 -> Matrix Concatenate/2
  Jacobian Jet3/1 -> Matrix Concatenate/3
  Jacobian Jet4/1 -> Matrix Concatenate/4
  "CoM6D -> CoMXYZ7"/1 -> J_CoM/1

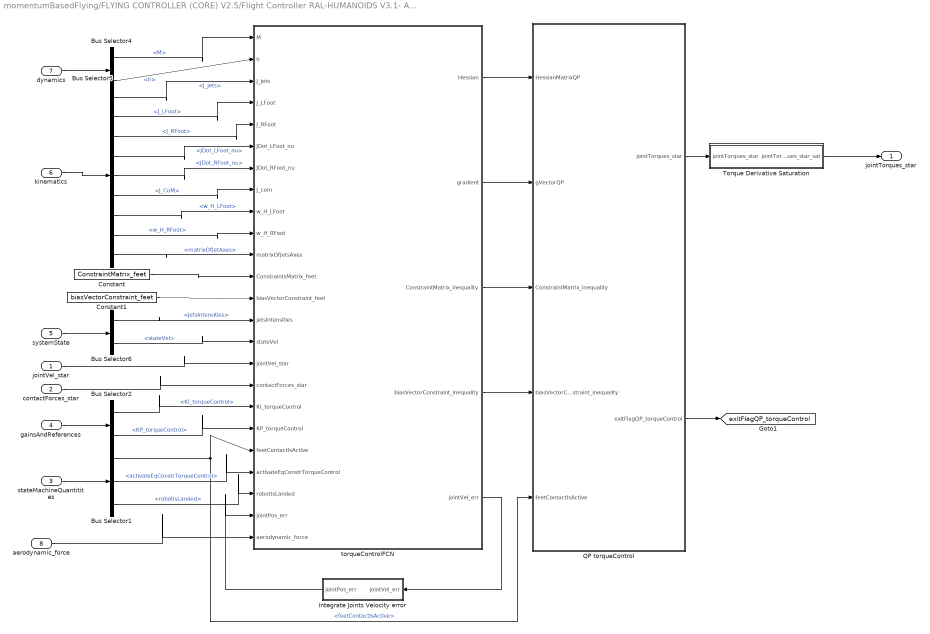
== system momentumBasedFlying/FLYING CONTROLLER (CORE) V2.5/Flight Controller RAL-HUMANOIDS V3.1- Aerodynamic Effects Compensation/Joint Torque Control for Flying ==
  jointVel_star : Inport
  contactForces_star : Inport  Port=2
  stateMachineQuantitites : Inport  Port=3
  gainsAndReferences : Inport  Port=4
  systemState : Inport  Port=5
  kinematics : Inport  Port=6
  dynamics : Inport  Port=7
  aerodynamic_force : Inport  Port=8
  Bus Selector1 : BusSelector  OutputSignals=feetContactIsActive,activateEqConstrTorqueControl,robotIsLanded
  Bus Selector2 : BusSelector  OutputSignals=KI_torqueControl,KP_torqueControl
  Bus Selector4 : BusSelector  OutputSignals=M,h
  Bus Selector5 : BusSelector  OutputSignals=J_jets,J_LFoot,J_RFoot,JDot_LFoot_nu,JDot_RFoot_nu,J_CoM,w_H_LFoot,w_H_RFoot,matrixOfJetAxes
  Bus Selector6 : BusSelector  OutputSignals=jetsIntensities,stateVel
  Constant : Constant  Value=ConstraintMatrix_feet
  Constant1 : Constant  Value=biasVectorConstraint_feet
  Integrate Joints Velocity error : Subsystem
  QP torqueControl : Subsystem
  Torque Derivative Saturation : Subsystem
  torqueControlFCN : MATLAB Function  TreatAsAtomicUnit=on
  jointTorques_star : Outport  VectorParamsAs1DForOutWhenUnconnected=off
  tag scope: exitFlagQP_torqueControl=global
  wires:
  Torque Derivative Saturation/1(jointTorques_star_sat) -> jointTorques_star/1
  Bus Selector1/2 -> torqueControlFCN/21(activateEqConstrTorqueControl)  "<activateEqConstrTorqueControl>"
  Bus Selector1/3 -> torqueControlFCN/22(robotIsLanded)  "<robotIsLanded>"
  torqueControlFCN/5(jointVel_err) -> Integrate Joints Velocity error/1(jointVel_err)
  Integrate Joints Velocity error/1(jointPos_err) -> torqueControlFCN/23(jointPos_err)
  Bus Selector5/9 -> torqueControlFCN/11(matrixOfJetsAxes)  "<matrixOfJetAxes>"
  jointVel_star/1 -> torqueControlFCN/16(jointVel_star)
  torqueControlFCN/4(biasVectorConstraint_inequality) -> QP torqueControl/4(biasVectorConstraint_inequality)
  torqueControlFCN/3(ConstraintMatrix_inequality) -> QP torqueControl/3(ConstraintMatrix_inequality)
  torqueControlFCN/2(gradient) -> QP torqueControl/2(gVectorQP)
  torqueControlFCN/1(Hessian) -> QP torqueControl/1(HessianMatrixQP)
  Bus Selector2/2 -> torqueControlFCN/19(KP_torqueControl)  "<KP_torqueControl>"
  Bus Selector2/1 -> torqueControlFCN/18(KI_torqueControl)  "<KI_torqueControl>"
  gainsAndReferences/1 -> Bus Selector2/1
  Bus Selector1/1 -> torqueControlFCN/20(feetContactIsActive), QP torqueControl/5(feetContactIsActive)  "<feetContactIsActive>"
  stateMachineQuantitites/1 -> Bus Selector1/1
  Bus Selector6/1 -> torqueControlFCN/14(jetsIntensities)  "<jetsIntensities>"
  QP torqueControl/2(exitFlagQP_torqueControl) -> [exitFlagQP_torqueControl]
  QP torqueControl/1(jointTorques_star) -> Torque Derivative Saturation/1(jointTorques_star)
  contactForces_star/1 -> torqueControlFCN/17(contactForces_star)
  Constant/1 -> torqueControlFCN/12(ConstraintsMatrix_feet)
  Constant1/1 -> torqueControlFCN/13(biasVectorConstraint_feet)
  Bus Selector5/8 -> torqueControlFCN/10(w_H_RFoot)  "<w_H_RFoot>"
  Bus Selector5/7 -> torqueControlFCN/9(w_H_LFoot)  "<w_H_LFoot>"
  Bus Selector5/5 -> torqueControlFCN/7(JDot_RFoot_nu)  "<JDot_RFoot_nu>"
  Bus Selector5/4 -> torqueControlFCN/6(JDot_LFoot_nu)  "<JDot_LFoot_nu>"
  Bus Selector5/3 -> torqueControlFCN/5(J_RFoot)  "<J_RFoot>"
  Bus Selector5/2 -> torqueControlFCN/4(J_LFoot)  "<J_LFoot>"
  Bus Selector5/1 -> torqueControlFCN/3(J_jets)  "<J_jets>"
  Bus Selector4/2 -> torqueControlFCN/2(h)  "<h>"
  Bus Selector4/1 -> torqueControlFCN/1(M)  "<M>"
  kinematics/1 -> Bus Selector5/1
  systemState/1 -> Bus Selector6/1
  dynamics/1 -> Bus Selector4/1
  Bus Selector6/2 -> torqueControlFCN/15(stateVel)  "<stateVel>"
  aerodynamic_force/1 -> torqueControlFCN/24(aerodynamic_force)
  Bus Selector5/6 -> torqueControlFCN/8(J_com)  "<J_CoM>"
